simulink model "example_CollectorEN12975conf"  (R2013b)
settings: Solver=ode45  StartTime=0.0  StopTime=24*3600  MaxStep=1800  RelTol=1e-3
libraries: carnot x10
settings Model: Creator=drhf  LastModifiedBy=drhf
settings OptimizationCC: ExpressionDepthLimit=2147483647
settings DebuggingCC: StateNameClashWarn=warning
settings GRTTargetCC: CombineOutputUpdateFcns=off  GRTInterface=on

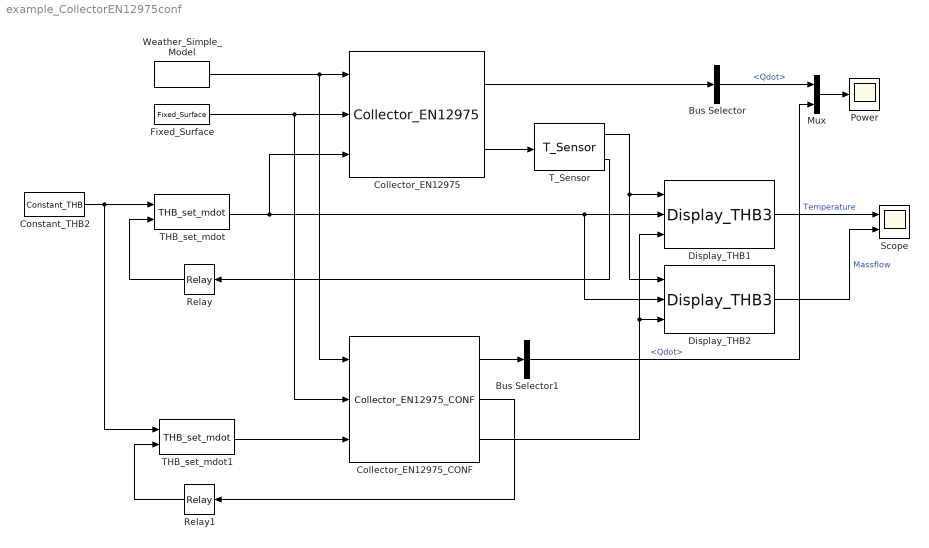
== system example_CollectorEN12975conf ==
  Bus Selector : BusSelector  OutputSignals=Qdot
  Bus Selector1 : BusSelector  OutputSignals=Qdot
  Collector_EN12975 : carnot/Source/Solar_Thermal/Collector_EN12975  acol=3.5  len=2.3  fta=0.8  c1=1.1  c2=0.001  c3=0  c4=0  c5=5000  c6=0  kblangle=[0:5:90]  KbL="[1.0000    1.0000    0.9999    0.9996    0.9991    0.9982    0.9965  0.9935    0.9886    0.9807    0.9678    0.9473    0.9148    0.8638   0.7846    0.6644    0.4907    0.2599    0.0000]"  kbtangle=[0:5:90]  KbT=[1.00000 1.00000 1.00000 1.00000 1.00000 1.00000 1.00000 1.00000 1.00000 1.00000 1.00000 0.87500 0.75000 0.62500 0.50000 0.37500 0.25000 0.12500 0]  Kd=0.92  lin=0  qua=0  tini=20
  Collector_EN12975_CONF : carnot/Source/Solar_Thermal/Collector_EN12975_CONF  parameterfile=DefaultCollector  tini=20  Ncollector=1
  Constant_THB2 : carnot/Source/Simple/Constant_THB  t=40  mdot=100/3600  p=1e5  mID=No Pressure Drop  fluid=Water  mix=0  dia=0.02  hgt=0
  Display_THB1 : carnot/Outputs/Display_THB3  t=on  m=off  p=off  id=off  mix=off  d=off
  Display_THB2 : carnot/Outputs/Display_THB3  t=off  m=on  p=off  id=off  mix=off  d=off
  Fixed_Surface : carnot/Weather/Fixed_Surface  colangle=30  colazi=0  colrot=0
  Mux : Mux  Inputs=2
  Power : Scope
  Relay : Relay  OnSwitchValue=47  OffSwitchValue=42  OnOutputValue=50/3600
  Relay1 : Relay  OnSwitchValue=47  OffSwitchValue=42  OnOutputValue=50/3600
  Scope : Scope  NumInputPorts=2
      settings: YMin=-5~-5  YMax=5~5
  THB_set_mdot : carnot/Source/Simple/THB_set_mdot
  THB_set_mdot1 : carnot/Source/Simple/THB_set_mdot
  T_Sensor : carnot/Control/T_Sensor  tc=10  t0=20
  Weather_Simple_Model : carnot/Weather/Weather_Simple_Model  lat=60  Ibn=900  Idg=100  tamb=5  deltaTsky=-6  rh=50  precip="10e-3/24/3600           % 10 mm in 24 h"  cloud=0.125  p=1013e2  vw=1  wdir=270
  wires:
  Weather_Simple_Model/1 -> Collector_EN12975/1, Collector_EN12975_CONF/1
  Fixed_Surface/1 -> Collector_EN12975/2, Collector_EN12975_CONF/2
  THB_set_mdot/1 -> Display_THB1/2, Display_THB2/2, Collector_EN12975/3
  Display_THB1/1 -> Scope/1  "Temperature"
  Collector_EN12975/1 -> Bus Selector/1
  Collector_EN12975_CONF/1 -> Bus Selector1/1
  Bus Selector/1 -> Mux/1  "<Qdot>"
  Bus Selector1/1 -> Mux/2  "<Qdot>"
  Mux/1 -> Power/1
  Constant_THB2/1 -> THB_set_mdot/1, THB_set_mdot1/1
  THB_set_mdot1/1 -> Collector_EN12975_CONF/3
  Collector_EN12975_CONF/3 -> Display_THB1/3, Display_THB2/3
  Collector_EN12975/2 -> T_Sensor/1
  T_Sensor/2 -> Relay/1
  Relay/1 -> THB_set_mdot/2
  Collector_EN12975_CONF/2 -> Relay1/1
  Relay1/1 -> THB_set_mdot1/2
  T_Sensor/1 -> Display_THB1/1, Display_THB2/1
  Display_THB2/1 -> Scope/2  "Massflow"
